simulink model "DTC_Vector_New"  (R2019b)
settings: Solver=ode4  StartTime=0.0  StopTime=1  FixedStep=50e-6  RelTol=1e-3
values from neighbouring files (symbols this model uses):
  B = 0    [Parameters_MPC.m]
  J = 0.0165    [Parameters_MPC.m]
  kr = (Lm/Lr)    (= 0.960714285714)    [Parameters_MPC.m]
  Lm = 0.0538    [Parameters_MPC.m]
  P = 2    [Parameters_MPC.m]
  r_sigma = Rs+Rr*(kr^2)    (= 0.445903864796)    [Parameters_MPC.m]
  Rs = 0.277    [Parameters_MPC.m]
  set_speed = 500    [Parameters_MPC.m]
  t_sigma = (sigma*Ls)/(r_sigma)    (= 0.00810392489023)    [Parameters_MPC.m]
  tr = Lr/Rr    (= 0.306010928962)    [Parameters_MPC.m]
libraries: powerlib_meascontrol x3, simulink x2, eeAsmDirectTorqueControl x1, powerlib x1
settings Model: Creator=91913  LastModifiedBy=91913
settings SolverCC: AlgebraicLoopSolver=LineSearch
settings DataIOCC: SaveOutput=off  DSMLogging=off  ReturnWorkspaceOutputs=off

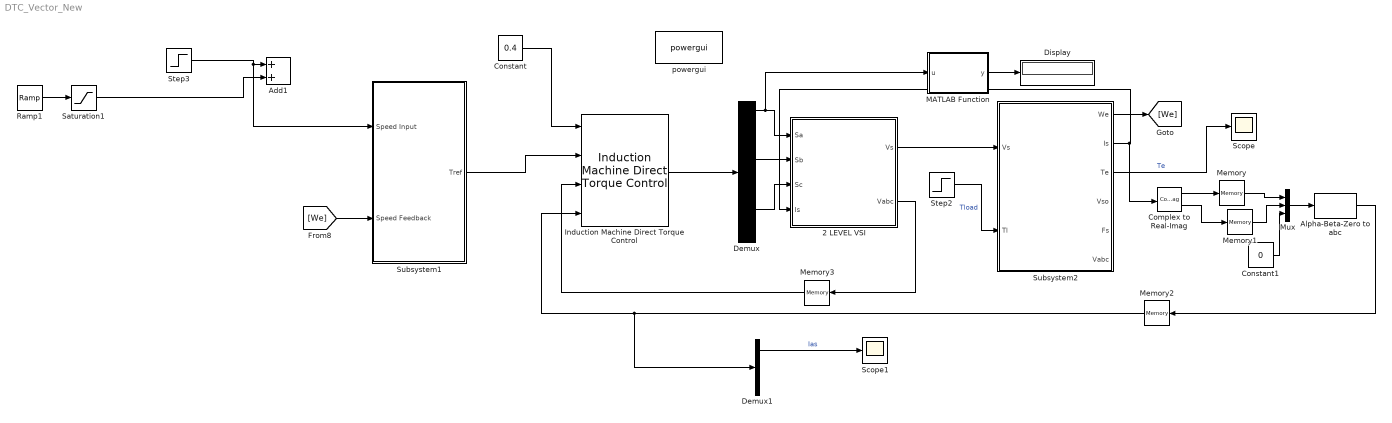
== system DTC_Vector_New ==
  2 LEVEL VSI : Subsystem
  Add1 : Sum
  Alpha-Beta-Zero to abc : powerlib_meascontrol/Transformations/Alpha-Beta-Zero to abc
      settings: SourceProductName=Simscape Electrical  SourceProductBaseCode=PS
  Complex to Real-Imag : ComplexToRealImag
  Constant : Constant  Value=0.4
  Constant1 : Constant  Value=0
  Demux : Demux  Outputs=6
  Demux1 : Demux  Outputs=3
  Display : Display
  Induction Machine Direct Torque Control : eeAsmDirectTorqueControl/Induction Machine Direct Torque Control  Rs=Rs  p=2  FluxHystBand=0.02  THystBand=2  Ts=-1
      settings: SourceProductName=Simscape Electrical  SourceProductBaseCode=PS
  MATLAB Function : MATLAB Function  TreatAsAtomicUnit=on
  Memory{,1..3} (4 alike) : Memory
  Mux : Mux  Inputs=3
  Ramp1 : simulink/Sources/Ramp  slope=-2*set_speed  start=0.4  InitialOutput=0
  Saturation1 : Saturate  UpperLimit=0  LowerLimit=-200
  Scope : Scope
  Scope1 : Scope
  Step2 : Step  Time=0.5  After=20  SampleTime=0
  Step3 : Step  Time=0.1  After=set_speed  SampleTime=0
  Subsystem1 : Subsystem
  Subsystem2 : Subsystem
  powergui : powerlib/powergui  Priority=1  SimulationMode=Continuous  SampleTime=50e-6  frequency=60  Iterations=50  frequencyindice=60  Pbase=100e6  ErrMax=1e-4  UnitsV=kV  UnitsW=MW  buscounter=0  FunctionMessages=off  echomessages=off  EnableUseOfTLC=off  CurrentSourceSwitches=off  DisableSnubberDevices=off  DisableRonSwitches=off  DisableVfSwitches=off  DisplayEquations=off  AutomaticDiscreteSolvers=off  SolverType=Tustin/Backward Euler (TBE)  Interpol=off  ExternalGateDelay=off  methode=off  Ts=100  x0status=blocks  SPID=on  SwTol=0  HookPort=off  NonlinearTolerance=1e-4  nMaxIteration=100  ContinueOnMaxIteration=off  RestoreLinks=warning  ResistiveCurrentMeasurement=off  Frange=[0:2:500]  Ylog=off  Xlog=on  ShowGrid=off  save=off  variable=ZData  structure=logsout  ZoomFFT=off  StartTime=1.5  cycles=40  DisplayStyle=1  fundamental=10.94  FreqAxis=on  MaxFrequency=1000  frequencyindicesteady=1  RmsSteady=1  display=off
      settings: SourceProductName=Simscape Electrical
  wires:
  [We] -> Subsystem1/2(Speed Feedback)
  Constant/1 -> Induction Machine Direct Torque Control/1
  Induction Machine Direct Torque Control/1 -> Demux/1
  Demux/1 -> MATLAB Function/1(u), 2 LEVEL VSI/1(Sa)
  Demux/3 -> 2 LEVEL VSI/2(Sb)
  Demux/5 -> 2 LEVEL VSI/3(Sc)
  2 LEVEL VSI/1(Vs) -> Subsystem2/1(Vs)
  Subsystem2/1(We) -> [We]
  Subsystem2/2(Is) -> Complex to Real-Imag/1, 2 LEVEL VSI/4(Is)
  Constant1/1 -> Mux/3
  Mux/1 -> Alpha-Beta-Zero to abc/1
  Complex to Real-Imag/1 -> Memory/1
  Memory/1 -> Mux/1
  Complex to Real-Imag/2 -> Memory1/1
  Memory1/1 -> Mux/2
  Alpha-Beta-Zero to abc/1 -> Memory2/1
  Memory2/1 -> Demux1/1, Induction Machine Direct Torque Control/4
  2 LEVEL VSI/2(Vabc) -> Memory3/1
  Memory3/1 -> Induction Machine Direct Torque Control/3
  Subsystem2/3(Te) -> Scope/1  "Te"
  Step2/1 -> Subsystem2/2(Tl)  "Tload"
  Demux1/1 -> Scope1/1  "Ias"
  Subsystem1/1(Tref) -> Induction Machine Direct Torque Control/2
  MATLAB Function/1(y) -> Display/1
  Step3/1 -> Subsystem1/1(Speed Input), Add1/1
  Saturation1/1 -> Add1/2
  Ramp1/1 -> Saturation1/1

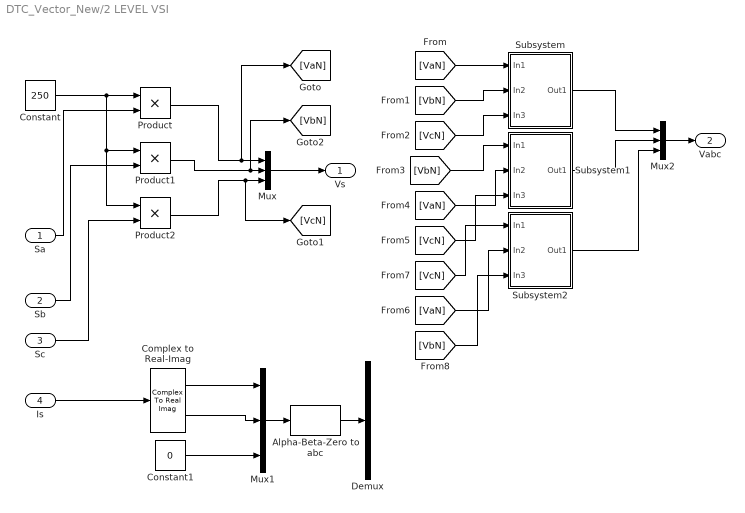
== system DTC_Vector_New/2 LEVEL VSI ==
  Sa : Inport
  Sb : Inport  Port=2
  Sc : Inport  Port=3
  Is : Inport  Port=4
  Alpha-Beta-Zero to abc : powerlib_meascontrol/Transformations/Alpha-Beta-Zero to abc
      settings: SourceProductName=Simscape Electrical  SourceProductBaseCode=PS
  Complex to Real-Imag : ComplexToRealImag
  Constant : Constant  Value=250
  Constant1 : Constant  Value=0
  Demux : Demux  Outputs=3
  Mux : Mux  Inputs=3
  Mux1 : Mux  Inputs=3
  Mux2 : Mux  Inputs=3
  Product : Product
  Product1 : Product
  Product2 : Product
  Subsystem : Subsystem
  Subsystem1 : Subsystem
  Subsystem2 : Subsystem
  Vs : Outport
  Vabc : Outport  Port=2
  wires:
  Sa/1 -> Product/2
  Sb/1 -> Product1/2
  Sc/1 -> Product2/2
  Constant/1 -> Product2/1, Product1/1, Product/1
  Product/1 -> [VaN], Mux/1
  Product1/1 -> [VbN], Mux/2
  Product2/1 -> [VcN], Mux/3
  Mux/1 -> Vs/1
  Alpha-Beta-Zero to abc/1 -> Demux/1
  Complex to Real-Imag/1 -> Mux1/1
  Complex to Real-Imag/2 -> Mux1/2
  Constant1/1 -> Mux1/3
  Mux1/1 -> Alpha-Beta-Zero to abc/1
  Is/1 -> Complex to Real-Imag/1
  [VaN] -> Subsystem/1(In1)
  [VbN] -> Subsystem/2(In2)
  [VcN] -> Subsystem/3(In3)
  [VbN] -> Subsystem1/1(In1)
  [VaN] -> Subsystem1/2(In2)
  [VcN] -> Subsystem1/3(In3)
  [VcN] -> Subsystem2/1(In1)
  [VaN] -> Subsystem2/2(In2)
  [VbN] -> Subsystem2/3(In3)
  Subsystem/1(Out1) -> Mux2/1
  Subsystem1/1(Out1) -> Mux2/2
  Subsystem2/1(Out1) -> Mux2/3
  Mux2/1 -> Vabc/1

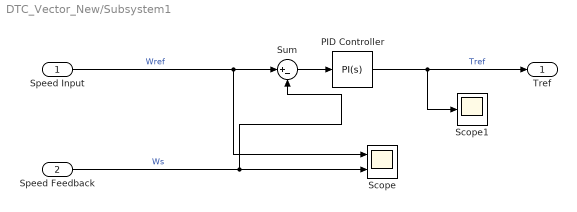
== system DTC_Vector_New/Subsystem1 ==
  Speed Input : Inport
  Speed Feedback : Inport  Port=2
  PID Controller : simulink/Continuous/PID Controller  Controller=PI  Form=Parallel  TimeDomain=Continuous-time  SampleTime=-1  IntegratorMethod=Forward Euler  FilterMethod=Forward Euler  ControllerParametersSource=internal  P=100  I=2000  D=0  UseFilter=on  N=100  TunerSelectOption=Transfer Function Based (PID Tuner App)  InitialConditionSource=internal  InitialConditionForIntegrator=0  InitialConditionForFilter=0  DifferentiatorICPrevScaledInput=0  ExternalReset=none  TrackingMode=off  Kt=1  LimitOutput=on  UpperSaturationLimit=30  LowerSaturationLimit=-30  LinearizeAsGain=on  AntiWindupMode=clamping  Kb=1  POutMin=[]  POutMax=[]  IOutMin=[]  IOutMax=[]  DOutMin=[]  DOutMax=[]  NOutMin=[]  NOutMax=[]  SumOutMin=[]  SumOutMax=[]  SaturationOutMin=[]  SaturationOutMax=[]  PParamMin=[]  PParamMax=[]  IParamMin=[]  IParamMax=[]  DParamMin=[]  DParamMax=[]  NParamMin=[]  NParamMax=[]  KbParamMin=[]  KbParamMax=[]  KtParamMin=[]  KtParamMax=[]  KbOutMin=[]  KbOutMax=[]  KtOutMin=[]  KtOutMax=[]  IntegratorOutMin=[]  IntegratorOutMax=[]  FilterOutMin=[]  FilterOutMax=[]  SumI1OutMin=[]  SumI1OutMax=[]  SumI2OutMin=[]  SumI2OutMax=[]  SumI3OutMin=[]  SumI3OutMax=[]  SumI4OutMin=[]  SumI4OutMax=[]  SumDOutMin=[]  SumDOutMax=[]  DifferentiatorOutMin=[]  DifferentiatorOutMax=[]  FilterDiffOutCoefMin=[]  FilterDiffOutCoefMax=[]  ReciprocalOutMin=[]  ReciprocalOutMax=[]  SumDenOutMin=[]  SumDenOutMax=[]  SumNumOutMin=[]  SumNumOutMax=[]  DivideOutMin=[]  DivideOutMax=[]  IntegratorContinuousStateAttributes=''  IntegratorStateMustResolveToSignalObject=off  IntegratorRTWStateStorageClass=Auto  FilterContinuousStateAttributes=''  FilterStateMustResolveToSignalObject=off  FilterRTWStateStorageClass=Auto  ParallelPVariant=InternalParameters  IdealPVariant=Disabled  IVariant=InternalParameters  DVariant=Disabled  IntegratorVariant=Continuous  SatVariant=Enabled  AWVariant=ContClampingParallel  PCopyVariant=Disabled  TRVariant=Disabled  FdbkBlocksVariant=Forward  IdealPFdbkVariant=Disabled  SatFdbkVariant=Disabled  DerivativeFilterVariant=Disabled  NVariant=Disabled  NCopyVariant=Disabled_SignalSpec  FilterICVariant=Disabled  IntegratorICVariant=InternalICs  ExternalResetVariant=Disabled  TRSumVariant=Passthrough  SumFdbkVariant=Disabled  SumVariant=Sum_PI
  Scope : Scope  NumInputPorts=2
  Scope1 : Scope
  Sum : Sum  Inputs=|+-
  Tref : Outport
  wires:
  Speed Input/1 -> Scope/1, Sum/1  "Wref"
  Sum/1 -> PID Controller/1
  PID Controller/1 -> Tref/1, Scope1/1  "Tref"
  Speed Feedback/1 -> Sum/2, Scope/2  "Ws"

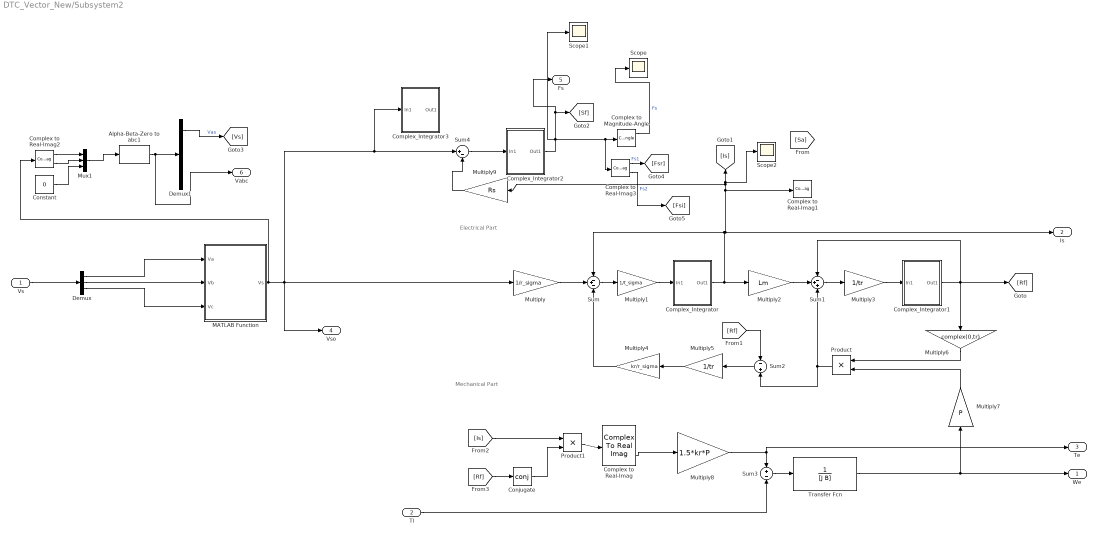
== system DTC_Vector_New/Subsystem2 ==
  note: Mechanical Part
  note: Electrical Part
  Vs : Inport
  Tl : Inport  Port=2
  Alpha-Beta-Zero to abc1 : powerlib_meascontrol/Transformations/Alpha-Beta-Zero to abc
      settings: SourceProductName=Simscape Electrical  SourceProductBaseCode=PS
  Complex to Magnitude-Angle : ComplexToMagnitudeAngle
  Complex to Real-Imag{,1..3} (4 alike) : ComplexToRealImag
  Complex_Integrator : Subsystem
  Complex_Integrator1 : Subsystem
  Complex_Integrator2 : Subsystem
  Complex_Integrator3 : Subsystem
  Conjugate : Math  Operator=conj  RndMeth=Zero  SaturateOnIntegerOverflow=on
  Constant : Constant  Value=0
  Demux : Demux  Outputs=3
  Demux1 : Demux  Outputs=3
  MATLAB Function : MATLAB Function  TreatAsAtomicUnit=on
  Multiply : Gain  Gain=1/r_sigma
  Multiply1 : Gain  Gain=1/t_sigma
  Multiply2 : Gain  Gain=Lm
  Multiply3 : Gain  Gain=1/tr
  Multiply4 : Gain  Gain=kr/r_sigma
  Multiply5 : Gain  Gain=1/tr
  Multiply6 : Gain  Gain=complex(0,tr)
  Multiply7 : Gain  Gain=P
  Multiply8 : Gain  Gain=1.5*kr*P
  Multiply9 : Gain  Gain=Rs
  Mux1 : Mux  Inputs=3
  Product : Product
  Product1 : Product
  Scope : Scope
  Scope1 : Scope
  Scope2 : Scope
  Sum : Sum  Inputs=-+-
  Sum1 : Sum  Inputs=-++
  Sum2 : Sum  Inputs=-+
  Sum3 : Sum  Inputs=+-
  Sum4 : Sum  Inputs=|+-
  Transfer Fcn : TransferFcn  Denominator=[J B]
  We : Outport
  Is : Outport  Port=2
  Te : Outport  Port=3
  Vso : Outport  Port=4
  Fs : Outport  Port=5
  Vabc : Outport  Port=6
  wires:
  [Is] -> Product1/1
  Multiply1/1 -> Complex_Integrator/1(In1)
  Multiply4/1 -> Sum/3
  Multiply3/1 -> Complex_Integrator1/1(In1)
  Sum1/1 -> Multiply3/1
  Complex to Real-Imag/2 -> Multiply8/1
  Complex_Integrator1/1(Out1) -> Sum1/1, [Rf], Multiply6/1
  Tl/1 -> Sum3/2
  Conjugate/1 -> Product1/2
  Multiply7/1 -> Product/2
  Multiply8/1 -> Sum3/1, Te/1
  Multiply2/1 -> Sum1/2
  Multiply/1 -> Sum/2
  Multiply6/1 -> Product/1
  Product/1 -> Sum2/2, Sum1/3
  Multiply5/1 -> Multiply4/1
  Sum2/1 -> Multiply5/1
  Transfer Fcn/1 -> We/1, Multiply7/1
  Sum/1 -> Multiply1/1
  [Rf] -> Conjugate/1
  Product1/1 -> Complex to Real-Imag/1
  Sum3/1 -> Transfer Fcn/1
  [Rf] -> Sum2/1
  Sum4/1 -> Complex_Integrator2/1(In1)
  Complex_Integrator2/1(Out1) -> Complex to Real-Imag3/1, Complex to Magnitude-Angle/1, Scope1/1, Fs/1, [Sf]
  Multiply9/1 -> Sum4/2
  Complex_Integrator/1(Out1) -> Multiply2/1, Multiply9/1, Scope2/1, [Is], Complex to Real-Imag1/1, Is/1, Sum/1
  MATLAB Function/1(Vs) -> Complex to Real-Imag2/1, Vso/1, Multiply/1, Complex_Integrator3/1(In1), Sum4/1
  Vs/1 -> Demux/1
  Demux/1 -> MATLAB Function/1(Va)
  Demux/2 -> MATLAB Function/2(Vb)
  Demux/3 -> MATLAB Function/3(Vc)
  Constant/1 -> Mux1/3
  Alpha-Beta-Zero to abc1/1 -> Vabc/1, Demux1/1
  Mux1/1 -> Alpha-Beta-Zero to abc1/1
  Complex to Real-Imag2/2 -> Mux1/2
  Complex to Real-Imag2/1 -> Mux1/1
  Demux1/1 -> [Vs]  "Vas"
  Complex to Magnitude-Angle/1 -> Scope/1  "Fs"
  Complex to Real-Imag3/1 -> [Fsr]  "Fs1"
  Complex to Real-Imag3/2 -> [Fsi]  "Fs2"

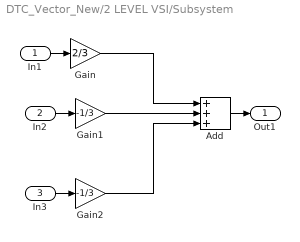
== system DTC_Vector_New/2 LEVEL VSI/Subsystem ==
  In1 : Inport
  In2 : Inport  Port=2
  In3 : Inport  Port=3
  Add : Sum  Inputs=3
  Gain : Gain  Gain=2/3
  Gain1 : Gain  Gain=-1/3
  Gain2 : Gain  Gain=-1/3
  Out1 : Outport
  wires:
  Gain2/1 -> Add/3
  In1/1 -> Gain/1
  Add/1 -> Out1/1
  Gain1/1 -> Add/2
  In2/1 -> Gain1/1
  Gain/1 -> Add/1
  In3/1 -> Gain2/1

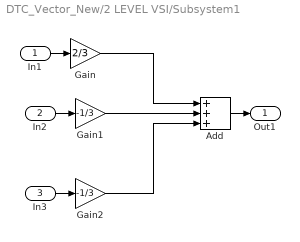
== system DTC_Vector_New/2 LEVEL VSI/Subsystem1 ==
  In1 : Inport
  In2 : Inport  Port=2
  In3 : Inport  Port=3
  Add : Sum  Inputs=3
  Gain : Gain  Gain=2/3
  Gain1 : Gain  Gain=-1/3
  Gain2 : Gain  Gain=-1/3
  Out1 : Outport
  wires:
  Gain2/1 -> Add/3
  In1/1 -> Gain/1
  Add/1 -> Out1/1
  Gain1/1 -> Add/2
  In2/1 -> Gain1/1
  Gain/1 -> Add/1
  In3/1 -> Gain2/1

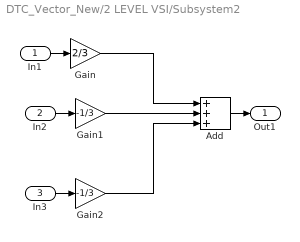
== system DTC_Vector_New/2 LEVEL VSI/Subsystem2 ==
  In1 : Inport
  In2 : Inport  Port=2
  In3 : Inport  Port=3
  Add : Sum  Inputs=3
  Gain : Gain  Gain=2/3
  Gain1 : Gain  Gain=-1/3
  Gain2 : Gain  Gain=-1/3
  Out1 : Outport
  wires:
  Gain2/1 -> Add/3
  In1/1 -> Gain/1
  Add/1 -> Out1/1
  Gain1/1 -> Add/2
  In2/1 -> Gain1/1
  Gain/1 -> Add/1
  In3/1 -> Gain2/1

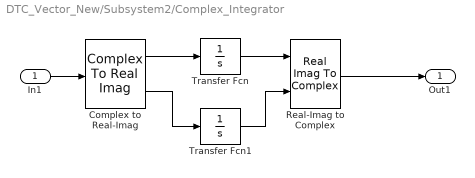
== system DTC_Vector_New/Subsystem2/Complex_Integrator ==
  In1 : Inport
  Complex to Real-Imag : ComplexToRealImag
  Real-Imag to Complex : RealImagToComplex
  Transfer Fcn : TransferFcn  Denominator=[1 0]
  Transfer Fcn1 : TransferFcn  Denominator=[1 0]
  Out1 : Outport
  wires:
  In1/1 -> Complex to Real-Imag/1
  Complex to Real-Imag/1 -> Transfer Fcn/1
  Complex to Real-Imag/2 -> Transfer Fcn1/1
  Transfer Fcn/1 -> Real-Imag to Complex/1
  Transfer Fcn1/1 -> Real-Imag to Complex/2
  Real-Imag to Complex/1 -> Out1/1

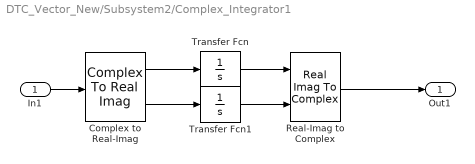
== system DTC_Vector_New/Subsystem2/Complex_Integrator1 ==
  In1 : Inport
  Complex to Real-Imag : ComplexToRealImag
  Real-Imag to Complex : RealImagToComplex
  Transfer Fcn : TransferFcn  Denominator=[1 0]
  Transfer Fcn1 : TransferFcn  Denominator=[1 0]
  Out1 : Outport
  wires:
  In1/1 -> Complex to Real-Imag/1
  Complex to Real-Imag/1 -> Transfer Fcn/1
  Complex to Real-Imag/2 -> Transfer Fcn1/1
  Transfer Fcn/1 -> Real-Imag to Complex/1
  Transfer Fcn1/1 -> Real-Imag to Complex/2
  Real-Imag to Complex/1 -> Out1/1

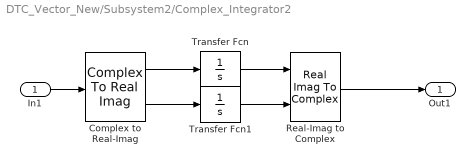
== system DTC_Vector_New/Subsystem2/Complex_Integrator2 ==
  In1 : Inport
  Complex to Real-Imag : ComplexToRealImag
  Real-Imag to Complex : RealImagToComplex
  Transfer Fcn : TransferFcn  Denominator=[1 0]
  Transfer Fcn1 : TransferFcn  Denominator=[1 0]
  Out1 : Outport
  wires:
  In1/1 -> Complex to Real-Imag/1
  Complex to Real-Imag/1 -> Transfer Fcn/1
  Complex to Real-Imag/2 -> Transfer Fcn1/1
  Transfer Fcn/1 -> Real-Imag to Complex/1
  Transfer Fcn1/1 -> Real-Imag to Complex/2
  Real-Imag to Complex/1 -> Out1/1

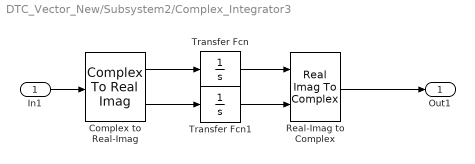
== system DTC_Vector_New/Subsystem2/Complex_Integrator3 ==
  In1 : Inport
  Complex to Real-Imag : ComplexToRealImag
  Real-Imag to Complex : RealImagToComplex
  Transfer Fcn : TransferFcn  Denominator=[1 0]
  Transfer Fcn1 : TransferFcn  Denominator=[1 0]
  Out1 : Outport
  wires:
  In1/1 -> Complex to Real-Imag/1
  Complex to Real-Imag/1 -> Transfer Fcn/1
  Complex to Real-Imag/2 -> Transfer Fcn1/1
  Transfer Fcn/1 -> Real-Imag to Complex/1
  Transfer Fcn1/1 -> Real-Imag to Complex/2
  Real-Imag to Complex/1 -> Out1/1

== matlab function DTC_Vector_New/Subsystem2/MATLAB Function ==
  data: Va input; Vs output; Vb input; Vc input
function Vs = fcn(Va,Vb,Vc)

a=complex(cos(2*pi/3),sin(2*pi/3)); 
Vs =(2/3)*(Va+(a*Vb)+((a^2)*Vc)) ;

== matlab function DTC_Vector_New/MATLAB Function ==
  data: u input; y output
function y = fcn(u)
persistent count prestate;
if(isempty(count))
    count=0;
end    
if(isempty(prestate))
    prestate=0;
end  
if(u~=prestate)
count=count+1;    
end
prestate=u;
y=count;
